simulink model "LOCAL_COMMUNICATIONS"  (R2021b)
settings: Solver=VariableStepAuto  StartTime=0.0  StopTime=inf  RelTol=1e-3
undefined symbols (not defined in the file): f
libraries: instrumentlib x7
settings Model: Creator=ccortes9  LastModifiedBy=ccortes9

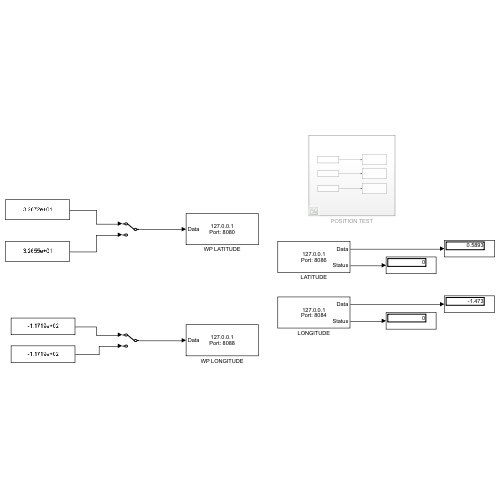
[thumbnail: Simulink's stored preview of the top-level diagram]
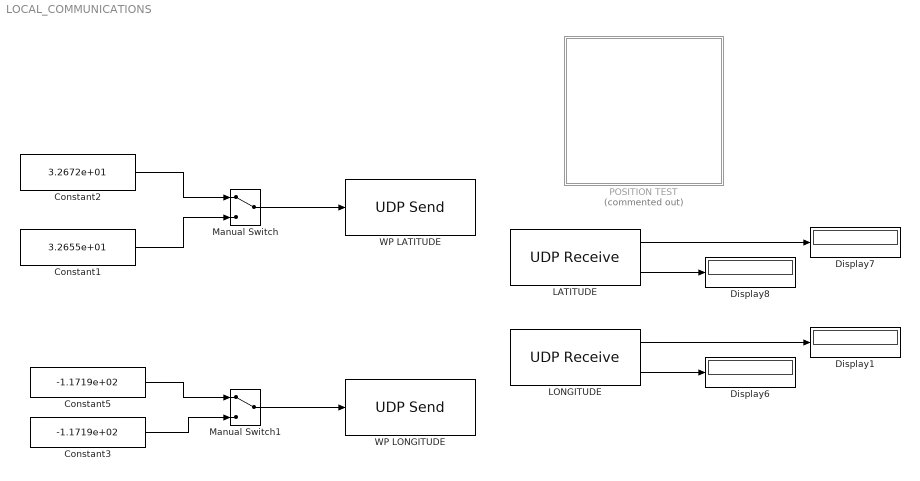
== system LOCAL_COMMUNICATIONS ==
  Constant1 : Constant  Value=3.2655e+01  SampleTime=0.03
  Constant2 : Constant  Value=3.2672e+01  SampleTime=0.03
  Constant3 : Constant  Value=-1.1719e+02  SampleTime=0.03
  Constant5 : Constant  Value=-1.1719e+02  SampleTime=0.03
  Display{1,6..8} (4 alike) : Display
  LATITUDE : instrumentlib/UDP Receive  Host=127.0.0.1  Port=8081  LocalPort=8086  EnablePortSharing=off  GetLatestData=off  DataSize=[1 1]  DataType=double  ASCIIFormatting=%f,  Terminator=LF  ByteOrder=BigEndian  EnableBlockingMode=off  Timeout=10  SampleTime=0.03  LocalAddress=127.0.0.1
  LONGITUDE : instrumentlib/UDP Receive  Host=127.0.0.1  Port=8083  LocalPort=8084  EnablePortSharing=off  GetLatestData=off  DataSize=[1 1]  DataType=double  ASCIIFormatting=%f,  Terminator=LF  ByteOrder=BigEndian  EnableBlockingMode=off  Timeout=10  SampleTime=0.03  LocalAddress=127.0.0.1
  Manual Switch : ManualSwitch
  Manual Switch1 : ManualSwitch
  POSITION TEST : Subsystem  Commented=on
  WP LATITUDE : instrumentlib/UDP Send  Host=127.0.0.1  Port=8080  LocalPort=8087  EnablePortSharing=off  ByteOrder=BigEndian  OutputDatagramPacketSize=512  EnableBlockingMode=on  LocalAddress=127.0.0.1
  WP LONGITUDE : instrumentlib/UDP Send  Host=127.0.0.1  Port=8088  LocalPort=8089  EnablePortSharing=off  ByteOrder=BigEndian  OutputDatagramPacketSize=512  EnableBlockingMode=on  LocalAddress=127.0.0.1
  wires:
  Constant2/1 -> Manual Switch/1
  Constant1/1 -> Manual Switch/2
  Constant5/1 -> Manual Switch1/1
  Constant3/1 -> Manual Switch1/2
  LONGITUDE/2 -> Display6/1
  LATITUDE/1 -> Display7/1
  LATITUDE/2 -> Display8/1
  LONGITUDE/1 -> Display1/1
  Manual Switch/1 -> WP LATITUDE/1
  Manual Switch1/1 -> WP LONGITUDE/1

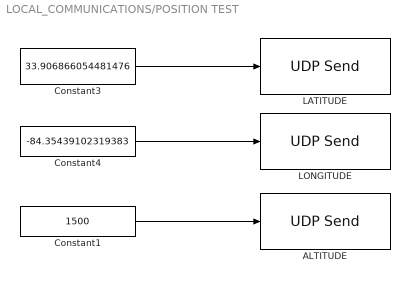
== system LOCAL_COMMUNICATIONS/POSITION TEST ==
  ALTITUDE : instrumentlib/UDP Send  Host=127.0.0.1  Port=8082  LocalPort=8085  EnablePortSharing=off  ByteOrder=BigEndian  OutputDatagramPacketSize=512  EnableBlockingMode=on  LocalAddress=127.0.0.1
  Constant1 : Constant  Value=1500  SampleTime=0.01
  Constant3 : Constant  Value=33.906866054481476  SampleTime=0.01
  Constant4 : Constant  Value=-84.35439102319383  SampleTime=0.01
  LATITUDE : instrumentlib/UDP Send  Host=127.0.0.1  Port=8086  LocalPort=8081  EnablePortSharing=off  ByteOrder=BigEndian  OutputDatagramPacketSize=512  EnableBlockingMode=on  LocalAddress=127.0.0.1
  LONGITUDE : instrumentlib/UDP Send  Host=127.0.0.1  Port=8084  LocalPort=8083  EnablePortSharing=off  ByteOrder=BigEndian  OutputDatagramPacketSize=512  EnableBlockingMode=on  LocalAddress=127.0.0.1
  wires:
  Constant4/1 -> LONGITUDE/1
  Constant1/1 -> ALTITUDE/1
  Constant3/1 -> LATITUDE/1
